simulink model "PMU"  (R2020a)
settings: Solver=VariableStepAuto  StartTime=0.0  StopTime=3  RelTol=1e-3
libraries: powerlib x7, simulink_extras x3, powerlib_meascontrol x1
settings Model: OrderedModelArguments=off  Creator=Chemes  LastModifiedBy=Madhura
settings DataIOCC: ReturnWorkspaceOutputs=off
settings DebuggingCC: SFMachineParentedDataDiag=error

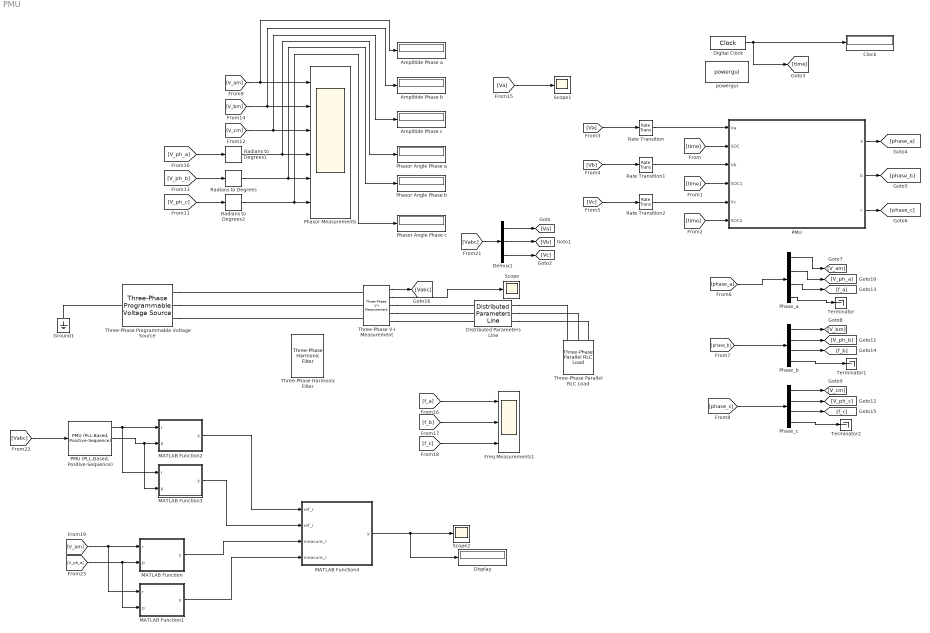
== system PMU ==
  Amplitide Phase a : Display
  Amplitide Phase b : Display
  Amplitide Phase c : Display
  Clock : Display
  Demux1 : Demux  Outputs=3
  Digital Clock : DigitalClock  SampleTime=1/50000
  Display : Display
  Distributed Parameters Line : powerlib/Elements/Distributed Parameters Line  Phases=3  Frequency=50  Resistance=[0.01273 0.3864]  Inductance="[0.9337e-3  4.1264e-3]"  Capacitance=[12.74e-9 7.751e-9]  Length=10  x1=[5.6843418860808e-14 281.691 281.691;314.159265358979 314.159265358979 314.159265358979;-0.0177670123217348 0.512763542316212 -1.05803278447868]  x2=[1.4210854715202e-14 274.972086644073 274.972086644073;314.159265358979 314.159265358979 314.159265358979;-1.58856333911663 0.33283657372806 -1.23795975306684]  x3=[1.09571086092759e-14 16.1582853427382 16.1582853427382;314.159265358979 314.159265358979 314.159265358979;-2.91438100278466 -2.81959274759355 1.89279623279113]  x4=[7.0866378270446e-15 18.197066930486 18.197066930486;314.159265358979 314.159265358979 314.159265358979;-1.58856333911663 0.33283657372806 -1.23795975306684]  x5=5.65541566995743e-05  V1=[5.684e-14 281.7 281.7;314.2 314.2 314.2;-0.01777 0.5128 -1.058]  V2=[1.421e-14 275 275;314.2 314.2 314.2;-1.589 0.3328 -1.238]  I1=[1.096e-14 16.16 16.16;314.2 314.2 314.2;-2.914 -2.82 1.893]  I2=[7.087e-15 18.2 18.2;314.2 314.2 314.2;-1.589 0.3328 -1.238]  nHarmo=1  Measurements=None
  Freq Measurements1 : Scope  NumInputPorts=3
  Ground1 : powerlib/Elements/Ground  LConnTagsString=a
  MATLAB Function : MATLAB Function  TreatAsAtomicUnit=on
  MATLAB Function1 : MATLAB Function  TreatAsAtomicUnit=on
  MATLAB Function2 : MATLAB Function  TreatAsAtomicUnit=on
  MATLAB Function3 : MATLAB Function  TreatAsAtomicUnit=on
  MATLAB Function4 : MATLAB Function  TreatAsAtomicUnit=on
  PMU : Subsystem
  "PMU (PLL-Based, Positive-Sequence)" : powerlib_meascontrol/Measurements/PMU (PLL-Based, Positive-Sequence)  nominalFrequency=50  samplingRate=64  reportingFactor=1
      settings: SourceProductBaseCode=PS
  Phase_a : Demux
  Phase_b : Demux
  Phase_c : Demux
  Phasor Angle Phase a : Display
  Phasor Angle Phase b : Display
  Phasor Angle Phase c : Display
  Phasor Measurements : Scope  NumInputPorts=6
  Radians to Degrees : simulink_extras/Transformations/Radians to Degrees
  Radians to Degrees1 : simulink_extras/Transformations/Radians to Degrees
  Radians to Degrees2 : simulink_extras/Transformations/Radians to Degrees
  Rate Transition : RateTransition  OutPortSampleTime=1/50000
  Rate Transition1 : RateTransition  OutPortSampleTime=1/50000
  Rate Transition2 : RateTransition  OutPortSampleTime=1/50000
  Scope : Scope
  Scope1 : Scope
  Scope2 : Scope
  Terminator : Terminator
  Terminator1 : Terminator
  Terminator2 : Terminator
  Three-Phase Harmonic Filter : powerlib/Elements/Three-Phase Harmonic Filter  LConnTagsString=A|B|C  RConnTagsString=n  FilterType=Double-tuned  FilterConnection=Y (neutral)  ParNom=[400 50]  Qc=49e6  Fr=[5*60]  Frd=[11*60 13*60]  Q=16  Measurements=None
      settings: AttributesFormatString=\n  SourceProductBaseCode=PS
  Three-Phase Parallel RLC Load : powerlib/Elements/Three-Phase Parallel RLC Load  LConnTagsString=A|B|C  Configuration=Y (grounded)  NominalVoltage=400  Vabc=[1e3 1e3 1e3]  Vabcp=[1e3 1e3 1e3]  NominalFrequency=50  UnbalancedPower=off  ActivePower=10e3  InductivePower=100  CapacitivePower=100  Pabc=[10e3 9e3 11e3]  QLabc=[100 90 110]  QCabc=[100 90 110]  Pabcp=[10e3 9e3 11e3]  QLabcp=[100 90 110]  QCabcp=[100 90 110]  Measurements=None  LoadType=constant Z
  Three-Phase Programmable Voltage Source : powerlib/Electrical Sources/Three-Phase Programmable Voltage Source  PositiveSequence="[281.691  0 50]"  VariationEntity=Amplitude  VariationType=Table of time-amplitude pairs  VariationTypeAlt=Step  VariationStep=0.5  VariationRate=10  VariationMagnitude=0.3  VariationFrequency=2  VariationTiming=[1 2]  VariationPhaseA=on  Amplitudes=[1 1.2 1.0 0.8 1]  TimeValues=[0 1 1.5 2.3 2.5]  HarmonicGeneration=off  HarmonicA=[3 0.2 -25 0]  HarmonicB=[5 0.15 35 2]  Timing="[0.05  3]"  BusType=swing  Pref=0  Qref=0  Qmin=-inf  Qmax=inf
  Three-Phase V-I Measurement : powerlib/Measurements/Three-Phase V-I Measurement  VoltageMeasurement=phase-to-ground  SetLabelV=off  LabelV=Vabc  Vpu=off  VpuLL=off  CurrentMeasurement=yes  SetLabelI=off  LabelI=Iabc  Ipu=off  Pbase=100e6  Vbase=500e3  OutputType=Complex  PhasorSimulation=off  PSBequivalent=0
  powergui : powerlib/powergui  Priority=1  SimulationMode=Continuous  SampleTime=50e-6  frequency=60  Iterations=50  frequencyindice=0  Pbase=100e6  ErrMax=1e-4  UnitsV=kV  UnitsW=MW  buscounter=0  FunctionMessages=off  echomessages=off  EnableUseOfTLC=off  CurrentSourceSwitches=off  DisableSnubberDevices=off  DisableRonSwitches=off  DisableVfSwitches=off  DisplayEquations=off  AutomaticDiscreteSolvers=off  SolverType=Tustin/Backward Euler (TBE)  Interpol=off  ExternalGateDelay=off  methode=off  Ts=100  x0status=blocks  SPID=on  SwTol=0  HookPort=off  NonlinearTolerance=1e-4  nMaxIteration=100  ContinueOnMaxIteration=off  RestoreLinks=warning  ResistiveCurrentMeasurement=off  Frange=[0:2:500]  Ylog=off  Xlog=on  ShowGrid=off  save=off  variable=ZData  structure=Current  ZoomFFT=off  StartTime=1.505  cycles=20  DisplayStyle=1  fundamental=50  FreqAxis=off  MaxFrequency=1000  frequencyindicesteady=1  RmsSteady=1  display=off
  wires:
  Digital Clock/1 -> [time], Clock/1
  Demux1/1 -> [Va]
  Demux1/2 -> [Vb]
  Demux1/3 -> [Vc]
  [Vb] -> Rate Transition1/1
  [Vc] -> Rate Transition2/1
  Rate Transition/1 -> PMU/1(Va)
  Rate Transition1/1 -> PMU/3(Vb)
  Rate Transition2/1 -> PMU/5(Vc)
  [time] -> PMU/2(SOC)
  [time] -> PMU/4(SOC1)
  [time] -> PMU/6(SOC2)
  Three-Phase V-I Measurement/2 -> Scope/1
  PMU/1(a) -> [phase_a]
  PMU/3(c) -> [phase_c]
  PMU/2(b) -> [phase_b]
  [phase_a] -> Phase_a/1
  Phase_a/1 -> [V_am]
  Phase_a/2 -> [V_ph_a]
  [phase_c] -> Phase_c/1
  [phase_b] -> Phase_b/1
  Phase_b/1 -> [V_bm]
  Phase_b/2 -> [V_ph_b]
  Phase_c/1 -> [V_cm]
  Phase_c/2 -> [V_ph_c]
  Phase_a/3 -> [f_a]
  Phase_c/3 -> [f_c]
  Phase_b/3 -> [f_b]
  Phase_a/4 -> Terminator/1
  Phase_b/4 -> Terminator1/1
  Phase_c/4 -> Terminator2/1
  [V_am] -> Amplitide Phase a/1, Phasor Measurements/1
  [V_bm] -> Amplitide Phase b/1, Phasor Measurements/2
  [V_cm] -> Amplitide Phase c/1, Phasor Measurements/3
  [V_ph_a] -> Radians to Degrees1/1
  [V_ph_b] -> Radians to Degrees/1
  [V_ph_c] -> Radians to Degrees2/1
  [Va] -> Scope1/1
  Radians to Degrees/1 -> Phasor Measurements/5, Phasor Angle Phase b/1
  Radians to Degrees1/1 -> Phasor Angle Phase a/1, Phasor Measurements/4
  Radians to Degrees2/1 -> Phasor Angle Phase c/1, Phasor Measurements/6
  [Va] -> Rate Transition/1
  [f_a] -> Freq Measurements1/1
  [f_b] -> Freq Measurements1/2
  [f_c] -> Freq Measurements1/3
  Three-Phase V-I Measurement/1 -> [Vabc]
  [Vabc] -> Demux1/1
  [Vabc] -> "PMU (PLL-Based, Positive-Sequence)"/1
  [V_am] -> MATLAB Function1/1(r), MATLAB Function/1(r)
  [V_ph_a] -> MATLAB Function1/2(p), MATLAB Function/2(p)
  "PMU (PLL-Based, Positive-Sequence)"/1 -> MATLAB Function2/1(r), MATLAB Function3/1(r)
  "PMU (PLL-Based, Positive-Sequence)"/2 -> MATLAB Function3/2(p), MATLAB Function2/2(p)
  MATLAB Function2/1(y) -> MATLAB Function4/1(ref_r)
  MATLAB Function3/1(y) -> MATLAB Function4/2(ref_i)
  MATLAB Function/1(y) -> MATLAB Function4/3(measure_r)
  MATLAB Function1/1(y) -> MATLAB Function4/4(measure_i)
  MATLAB Function4/1(y) -> Display/1, Scope2/1
  connections:
  Three-Phase V-I Measurement/RConn1 -- Distributed Parameters Line/LConn1
  Three-Phase V-I Measurement/RConn2 -- Distributed Parameters Line/LConn2
  Three-Phase V-I Measurement/RConn3 -- Distributed Parameters Line/LConn3
  Distributed Parameters Line/RConn1 -- Three-Phase Parallel RLC Load/LConn1
  Distributed Parameters Line/RConn2 -- Three-Phase Parallel RLC Load/LConn2
  Distributed Parameters Line/RConn3 -- Three-Phase Parallel RLC Load/LConn3
  Three-Phase Programmable Voltage Source/RConn1 -- Three-Phase V-I Measurement/LConn1
  Three-Phase Programmable Voltage Source/RConn2 -- Three-Phase V-I Measurement/LConn2
  Three-Phase Programmable Voltage Source/RConn3 -- Three-Phase V-I Measurement/LConn3
  Ground1/LConn1 -- Three-Phase Programmable Voltage Source/LConn1

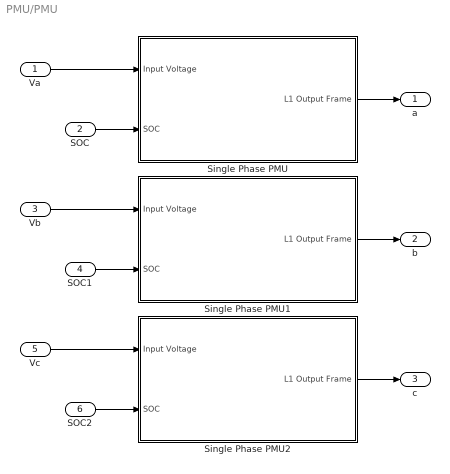
== system PMU/PMU ==
  Va : Inport
  SOC : Inport  Port=2
  Vb : Inport  Port=3
  SOC1 : Inport  Port=4
  Vc : Inport  Port=5
  SOC2 : Inport  Port=6
  Single Phase PMU : Subsystem  mask{Window_Length=2000, Nominal_Frequency=50, Signal_Sample_rate=50000, Frame_Rate=50, n_bins=8, P_Iter=3, Q_Iter=3, Threshold_rocof=[3, 25, 0.035], Lowpass_Coeff=[-0.5913, 0.2043, 0.2043 ], Buffer_Overlap=1, PhaseMode=Any frequency, TimeBase=second}
      mask prompts: Window_Length "Window Length (samples)"; Nominal_Frequency "Power Frequency (Hz)"; Signal_Sample_rate "Sample Rate (sample/s)"; Frame_Rate "Frame Rate (frame/s)"; n_bins "Number of DFT bins"; P_Iter "P (number of e-iter)"; Q_Iter "Q (number of i-iter)"; Threshold_rocof "Rocof Thresholds"; Lowpass_Coeff "Rocof Lowpass Filter Coeff"; Buffer_Overlap "Buffer Overlap (samples)"; PhaseMode "Phase Reference Mode"; TimeBase "Fracsec Time Base"
      mask TypeOptions PhaseMode: Nominal frequency only | Any frequency
      mask TypeOptions TimeBase: second | millisecond | microsecond | nanosecond
      mask DialogControl DescGroupVar Prompt: Phasor Measurment Unit
      mask DialogControl DescTextVar Prompt: This block calculates the following quantities of a Power System Signal: Frequency[Hz], Synchrophasor (RMS[V], Phase[rad]), Rocof [Hz/s], given an input signal and its correspondent timestamp data.
      mask DialogControl ParameterGroupVar Prompt: Basic Parameters
      mask DialogControl SystemParameters Prompt: System Parameters
  Single Phase PMU1 : Subsystem  mask{Window_Length=3000, Nominal_Frequency=50, Signal_Sample_rate=50000, Frame_Rate=100, n_bins=10, P_Iter=3, Q_Iter=3, Threshold_rocof=[3, 25, 0.035], Lowpass_Coeff=[-0.5913, 0.2043, 0.2043 ], Buffer_Overlap=1, PhaseMode=Any frequency, TimeBase=second}
      mask prompts: Window_Length "Window Length (samples)"; Nominal_Frequency "Power Frequency (Hz)"; Signal_Sample_rate "Sample Rate (sample/s)"; Frame_Rate "Frame Rate (frame/s)"; n_bins "Number of DFT bins"; P_Iter "P (number of e-iter)"; Q_Iter "Q (number of i-iter)"; Threshold_rocof "Rocof Thresholds"; Lowpass_Coeff "Rocof Lowpass Filter Coeff"; Buffer_Overlap "Buffer Overlap (samples)"; PhaseMode "Phase Reference Mode"; TimeBase "Fracsec Time Base"
      mask TypeOptions PhaseMode: Nominal frequency only | Any frequency
      mask TypeOptions TimeBase: second | millisecond | microsecond | nanosecond
      mask DialogControl DescGroupVar Prompt: Phasor Measurment Unit
      mask DialogControl DescTextVar Prompt: This block calculates the following quantities of a Power System Signal: Frequency[Hz], Synchrophasor (RMS[V], Phase[rad]), Rocof [Hz/s], given an input signal and its correspondent timestamp data.
      mask DialogControl ParameterGroupVar Prompt: Basic Parameters
      mask DialogControl SystemParameters Prompt: System Parameters
  Single Phase PMU2 : Subsystem  mask{Window_Length=3000, Nominal_Frequency=50, Signal_Sample_rate=50000, Frame_Rate=100, n_bins=10, P_Iter=3, Q_Iter=3, Threshold_rocof=[3, 25, 0.035], Lowpass_Coeff=[-0.5913, 0.2043, 0.2043 ], Buffer_Overlap=1, PhaseMode=Any frequency, TimeBase=second}
      mask prompts: Window_Length "Window Length (samples)"; Nominal_Frequency "Power Frequency (Hz)"; Signal_Sample_rate "Sample Rate (sample/s)"; Frame_Rate "Frame Rate (frame/s)"; n_bins "Number of DFT bins"; P_Iter "P (number of e-iter)"; Q_Iter "Q (number of i-iter)"; Threshold_rocof "Rocof Thresholds"; Lowpass_Coeff "Rocof Lowpass Filter Coeff"; Buffer_Overlap "Buffer Overlap (samples)"; PhaseMode "Phase Reference Mode"; TimeBase "Fracsec Time Base"
      mask TypeOptions PhaseMode: Nominal frequency only | Any frequency
      mask TypeOptions TimeBase: second | millisecond | microsecond | nanosecond
      mask DialogControl DescGroupVar Prompt: Phasor Measurment Unit
      mask DialogControl DescTextVar Prompt: This block calculates the following quantities of a Power System Signal: Frequency[Hz], Synchrophasor (RMS[V], Phase[rad]), Rocof [Hz/s], given an input signal and its correspondent timestamp data.
      mask DialogControl ParameterGroupVar Prompt: Basic Parameters
      mask DialogControl SystemParameters Prompt: System Parameters
  a : Outport
  b : Outport  Port=2
  c : Outport  Port=3
  wires:
  Single Phase PMU/1(L1 Output Frame) -> a/1
  Va/1 -> Single Phase PMU/1(Input Voltage)
  SOC/1 -> Single Phase PMU/2(SOC)
  Vc/1 -> Single Phase PMU2/1(Input Voltage)
  SOC2/1 -> Single Phase PMU2/2(SOC)
  Vb/1 -> Single Phase PMU1/1(Input Voltage)
  Single Phase PMU1/1(L1 Output Frame) -> b/1
  Single Phase PMU2/1(L1 Output Frame) -> c/1
  SOC1/1 -> Single Phase PMU1/2(SOC)

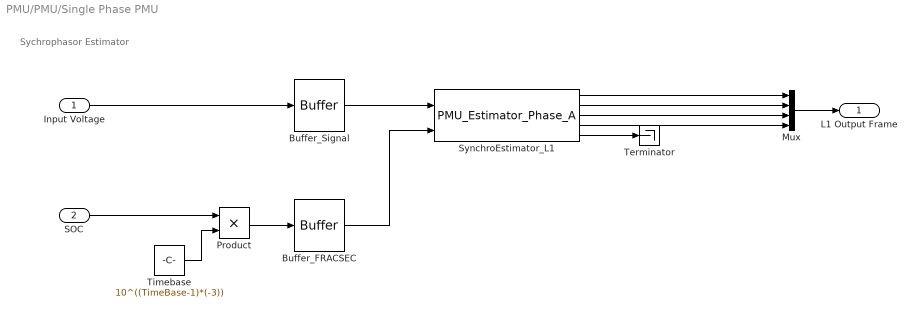
== system PMU/PMU/Single Phase PMU ==
  note: Sychrophasor Estimator
  Input Voltage : Inport
  SOC : Inport  Port=2
  Buffer_FRACSEC : Buffer  N=Window_Length  V=Window_Length-Buffer_Overlap  OutputFrames=off
  Buffer_Signal : Buffer  N=Window_Length  V=Window_Length-Buffer_Overlap  OutputFrames=off
  Mux : Mux
  Product : Product
  SynchroEstimator_L1 : S-Function  FunctionName=PMU_Estimator_Phase_A  Parameters=Signal_Sample_rate,Nominal_Frequency,Window_Length,P_Iter,Frame_Rate,PhaseMode, Threshold_rocof, Lowpass_Coeff,Q_Iter,n_bins  SFunctionDeploymentMode=off  EnableBusSupport=off
  Terminator : Terminator
  Timebase : Constant  Value=10^((TimeBase-1)*(-3))  SampleTime=Signal_Sample_rate
  L1 Output Frame : Outport
  wires:
  Mux/1 -> L1 Output Frame/1
  SynchroEstimator_L1/3 -> Mux/3
  SynchroEstimator_L1/4 -> Mux/4
  Buffer_Signal/1 -> SynchroEstimator_L1/1
  SOC/1 -> Product/1
  Timebase/1 -> Product/2
  SynchroEstimator_L1/2 -> Mux/2
  SynchroEstimator_L1/1 -> Mux/1
  Buffer_FRACSEC/1 -> SynchroEstimator_L1/2
  Input Voltage/1 -> Buffer_Signal/1
  Product/1 -> Buffer_FRACSEC/1
  SynchroEstimator_L1/5 -> Terminator/1

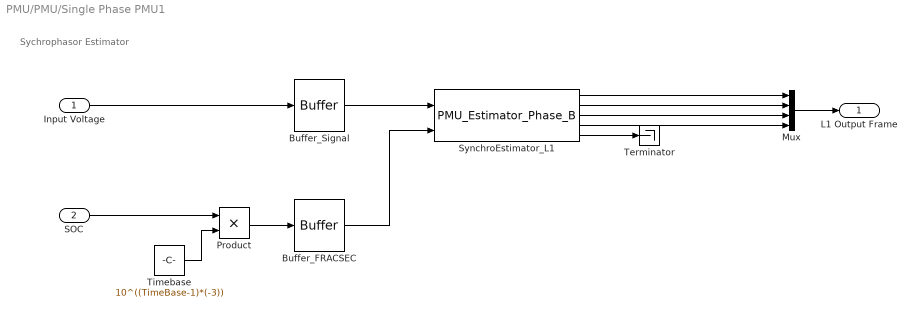
== system PMU/PMU/Single Phase PMU1 ==
  note: Sychrophasor Estimator
  Input Voltage : Inport
  SOC : Inport  Port=2
  Buffer_FRACSEC : Buffer  N=Window_Length  V=Window_Length-Buffer_Overlap  OutputFrames=off
  Buffer_Signal : Buffer  N=Window_Length  V=Window_Length-Buffer_Overlap  OutputFrames=off
  Mux : Mux
  Product : Product
  SynchroEstimator_L1 : S-Function  FunctionName=PMU_Estimator_Phase_B  Parameters=Signal_Sample_rate,Nominal_Frequency,Window_Length,P_Iter,Frame_Rate,PhaseMode, Threshold_rocof, Lowpass_Coeff,Q_Iter,n_bins  SFunctionDeploymentMode=off  EnableBusSupport=off
  Terminator : Terminator
  Timebase : Constant  Value=10^((TimeBase-1)*(-3))  SampleTime=Signal_Sample_rate
  L1 Output Frame : Outport
  wires:
  Mux/1 -> L1 Output Frame/1
  SynchroEstimator_L1/3 -> Mux/3
  SynchroEstimator_L1/4 -> Mux/4
  Buffer_Signal/1 -> SynchroEstimator_L1/1
  SOC/1 -> Product/1
  Timebase/1 -> Product/2
  SynchroEstimator_L1/2 -> Mux/2
  SynchroEstimator_L1/1 -> Mux/1
  Buffer_FRACSEC/1 -> SynchroEstimator_L1/2
  Input Voltage/1 -> Buffer_Signal/1
  Product/1 -> Buffer_FRACSEC/1
  SynchroEstimator_L1/5 -> Terminator/1

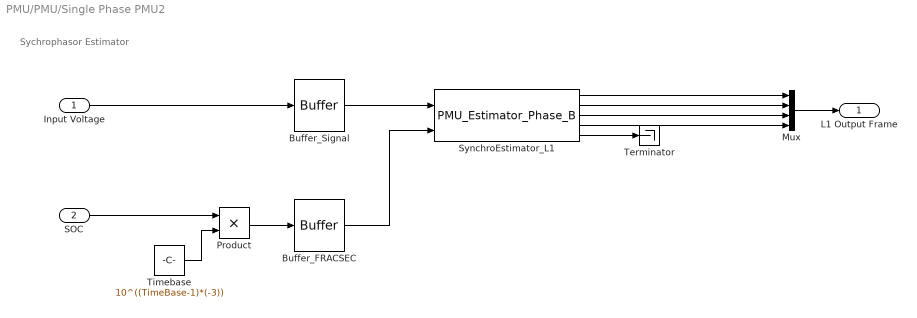
== system PMU/PMU/Single Phase PMU2 ==
  note: Sychrophasor Estimator
  Input Voltage : Inport
  SOC : Inport  Port=2
  Buffer_FRACSEC : Buffer  N=Window_Length  V=Window_Length-Buffer_Overlap  OutputFrames=off
  Buffer_Signal : Buffer  N=Window_Length  V=Window_Length-Buffer_Overlap  OutputFrames=off
  Mux : Mux
  Product : Product
  SynchroEstimator_L1 : S-Function  FunctionName=PMU_Estimator_Phase_B  Parameters=Signal_Sample_rate,Nominal_Frequency,Window_Length,P_Iter,Frame_Rate,PhaseMode, Threshold_rocof, Lowpass_Coeff,Q_Iter,n_bins  SFunctionDeploymentMode=off  EnableBusSupport=off
  Terminator : Terminator
  Timebase : Constant  Value=10^((TimeBase-1)*(-3))  SampleTime=Signal_Sample_rate
  L1 Output Frame : Outport
  wires:
  Mux/1 -> L1 Output Frame/1
  SynchroEstimator_L1/3 -> Mux/3
  SynchroEstimator_L1/4 -> Mux/4
  Buffer_Signal/1 -> SynchroEstimator_L1/1
  SOC/1 -> Product/1
  Timebase/1 -> Product/2
  SynchroEstimator_L1/2 -> Mux/2
  SynchroEstimator_L1/1 -> Mux/1
  Buffer_FRACSEC/1 -> SynchroEstimator_L1/2
  Input Voltage/1 -> Buffer_Signal/1
  Product/1 -> Buffer_FRACSEC/1
  SynchroEstimator_L1/5 -> Terminator/1

== matlab function PMU/MATLAB Function1 ==
  data: r input; y output; p input
function y = fcn(r, p)

y = r*tan(p)/(sqrt(1+(tan(p)^2)));

== matlab function PMU/MATLAB Function ==
  data: r input; y output; p input
function y = fcn(r, p)

y = r/(sqrt(1+(tan(p)^2)));

== matlab function PMU/MATLAB Function2 ==
  data: r input; y output; p input
function y = fcn(r, p)

y = r/(sqrt(1+(tan(p)^2)));

== matlab function PMU/MATLAB Function3 ==
  data: r input; y output; p input
function y = fcn(r, p)

y = r*tan(p)/(sqrt(1+(tan(p)^2)));

== matlab function PMU/MATLAB Function4 ==
  data: ref_r input; y output; ref_i input; measure_r input; measure_i input
function y = fcn(ref_r, ref_i, measure_r, measure_i)

y = (sqrt((((measure_r - ref_r)^2) + ((measure_i - ref_i)^2))/(((ref_r)^2) + ((ref_i)^2))));
